simulink model "AudioEcho"  (R2015a)
settings: Solver=ode45  StartTime=0.0  StopTime=90  RelTol=1e-3
libraries: dspvision x1, dspsnks4 x1
settings Model: Creator=ekulasek  LastModifiedBy=chulantha

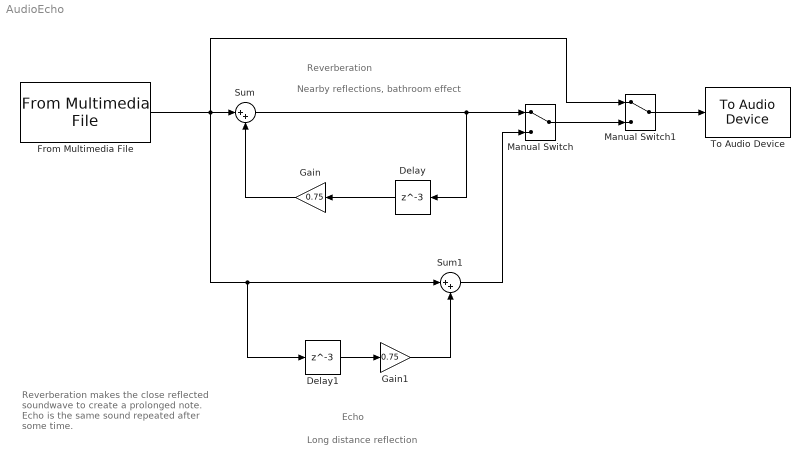
== system AudioEcho ==
  note: Reverberation makes the close
      | reflected soundwave to create a
      | prolonged note. Echo is the same sound
      | repeated after some time.
  note: Long distance reflection
  note: Nearby reflections, bathroom effect
  note: Echo
  note: Reverberation
  Delay : Delay  DelayLength=3  InitialCondition=0
  Delay1 : Delay  DelayLength=3  InitialCondition=0
  From Multimedia File : dspvision/From Multimedia File  inputFilename=/home/chulantha/Malabe/classes/SignalsAndSystems/Programs/song02.ogg  loop=on  numPlays=inf  outputStreams=Audio only  videoDataType=single  audioDataType=double  inheritSampleTime=on  userDefinedSampleTime=1/30  noAudioOutput=off  isIntensityVideo=off  fourcc=RGB  colorVideoFormat=Separate color signals  outputEOF=off  dataOrg=Column-major  audioFrameSize=1024  computeAudioFrameSize=off  outSamplingMode=Sample based
  Gain : Gain  Gain=0.75
  Gain1 : Gain  Gain=0.75
  Manual Switch : ManualSwitch
  Manual Switch1 : ManualSwitch
  Sum : Sum  Inputs=|++
  Sum1 : Sum  Inputs=|++
  To Audio Device : dspsnks4/To Audio Device  deviceName=Default  inheritSampleRate=on  sampleRate=44100  deviceDatatype=Determine from input data type  autoBufferSize=on  bufferSize=4096  queueDuration=1.0  defaultOutputChannelMapping=on  outputChannelMapping=1:2  outputNumUnderrunSamples=off
  wires:
  Gain/1 -> Sum/2
  Delay/1 -> Gain/1
  Sum/1 -> Manual Switch/1, Delay/1
  From Multimedia File/1 -> Manual Switch1/1, Delay1/1, Sum1/1, Sum/1
  Sum1/1 -> Manual Switch/2
  Delay1/1 -> Gain1/1
  Gain1/1 -> Sum1/2
  Manual Switch1/1 -> To Audio Device/1
  Manual Switch/1 -> Manual Switch1/2
